simulink model "5_model"  (R2014b)
settings: Solver=ode45  StartTime=0.0  StopTime=15.0  RelTol=1e-3
undefined symbols (not defined in the file): b, k, m
settings Model: Creator=Shane Reynolds  LastModifiedBy=Shane Reynolds

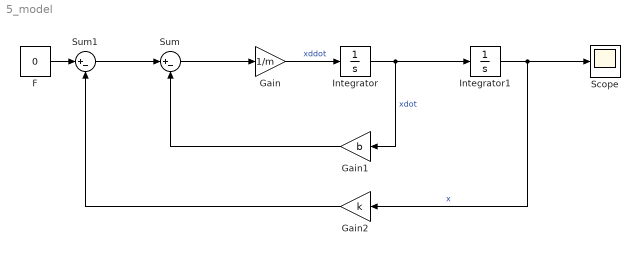
== system 5_model ==
  F : Constant  Value=0
  Gain : Gain  Gain=1/m
  Gain1 : Gain  Gain=b
  Gain2 : Gain  Gain=k
  Integrator : Integrator
  Integrator1 : Integrator  InitialCondition=10
  Scope : Scope
  Sum : Sum  Inputs=|+-
  Sum1 : Sum  Inputs=|+-
  wires:
  Gain/1 -> Integrator/1  "xddot"
  Integrator/1 -> Gain1/1, Integrator1/1  "xdot"
  Integrator1/1 -> Scope/1, Gain2/1  "x"
  Gain1/1 -> Sum/2
  Gain2/1 -> Sum1/2
  Sum1/1 -> Sum/1
  Sum/1 -> Gain/1
  F/1 -> Sum1/1
